simulink model "APA_AEB_Version_0_1"  (R2019a)
settings: Solver=FixedStepAuto  StartTime=0.0  StopTime=2  FixedStep=0.01  RelTol=1e-3
libraries: simulink x4, dspnetwork x1, autolibshared x1
(part 2 of 3)

== matlab function APA_AEB_Version_0_1/Ultarsonic Processment /Subsystem1/Subsystem1/MATLAB Function ==
  data: front_leftSide_uss_dist input single; front_leftFront_uss_dist input single; front_leftMiddle_uss_dist input single; front_rightMiddle_uss_dist input single; front_rightFront_uss_dist input single; front_rightSide_uss_dist input single; rear_leftSide_uss_dist input single; rear_leftRear_uss_dist input single; rear_leftMiddle_uss_dist input single; rear_rightMiddle_uss_dist input single; rear_rightRear_uss_dist input single; Useful_flag output single; Front_Object_dist_x output single; Front_Object_dist_y output single; Rear_Object_dist_x output single; Rear_Object_dist_y output single; rear_rightSide_uss_dist input single; USS_Position input single
function [ Useful_flag,Front_Object_dist_x,Front_Object_dist_y,Rear_Object_dist_x,Rear_Object_dist_y]  = Obj_Position_Identify(front_leftSide_uss_dist,...
                                        front_leftFront_uss_dist,...
                                        front_leftMiddle_uss_dist,...
                                        front_rightMiddle_uss_dist,...
                                        front_rightFront_uss_dist,...
                                        front_rightSide_uss_dist,...
                                        rear_leftSide_uss_dist,...
                                        rear_leftRear_uss_dist,...
                                        rear_leftMiddle_uss_dist,...
                                        rear_rightMiddle_uss_dist,...
                                        rear_rightRear_uss_dist,...
                                        rear_rightSide_uss_dist,...
                                        USS_Position)
                                    
        USS_dist  = [single(360.6744),single(640.6000),single(360.6231),single(398.5876),single(560.8000),single(398.5876)];
        %
        USS_ID  = [single(0),single(0),single(0),single(0),single(0),single(0),single(0),single(0),single(0),single(0),single(0),single(0)];
        %
        Front_leftSide_uss_position_x  = single(3237.1);
        %
        Front_leftSide_uss_position_y  = single(-913.1);
        %
        Front_leftFront_uss_position_x  = single(3528.8);
        %
        Front_leftFront_uss_position_y  = single(-650.5);
        %
        Front_leftMiddle_uss_position_x  = single(3673.9);
        %
        Front_leftMiddle_uss_position_y  = single(-320.3);
        %
        Front_rightMiddle_uss_position_x  = single(3673.9);
        %
        Front_rightMiddle_uss_position_y  = single(320.3);
        %
        Front_rightFront_uss_position_x  =  single(3528.7);
        %
        Front_rightFront_uss_position_y  =  single(650.4);
        %
        Front_rightSide_uss_position_x  =  single(3337.1);
        %
        Front_rightSide_uss_position_y  =  single(913.1);
        %
        Rear_leftSide_uss_position_x  =  single(-432.3);
        %
        Rear_leftSide_uss_position_y  =  single(-915.1);
        %
        Rear_leftRear_uss_position_x  =  single(-784.2);
        %
        Rear_leftRear_uss_position_y  =  single(-660.4);
        %
        Rear_leftMiddle_uss_position_x  =  single(-904.5);
        %
        Rear_leftMiddle_uss_position_y  =  single(-280.4);
        %
        Rear_rightMiddle_uss_position_x  =  single(-904.5);
        %
        Rear_rightMiddle_uss_position_y  =  single(280.4);
        %
        Rear_rightRear_uss_position_x  =  single(-784.2);
        %
        Rear_rightRear_uss_position_y  =  single(660.4);
        %
        Rear_rightSide_uss_position_x  =  single(-432.3);
        %
        Rear_rightSide_uss_position_y  =  single(915.1);
        %
        Front_Object_dist_x  = [single(0),single(0),single(0),single(0),single(0)];
        %
        Front_Object_dist_y  = [single(0),single(0),single(0),single(0),single(0)];
        %
        Rear_Object_dist_x  = [single(0),single(0),single(0),single(0),single(0)];
        %
        Rear_Object_dist_y  = [single(0),single(0),single(0),single(0),single(0)];
        %
        Left_Object_dist_x  = [single(0),single(0),single(0),single(0),single(0)];
        %
        Left_Object_dist_y  = [single(0),single(0),single(0),single(0),single(0)];
        %
        Right_Object_dist_x  = [single(0),single(0),single(0),single(0),single(0)];
        %
        Right_Object_dist_y  = [single(0),single(0),single(0),single(0),single(0)];
        %
        point_num  = single(5);
        %
        Front_leftSide_uss_FOV  = [single(0.9986),single(0.0523);single(0.0523),single(-0.9986)];
        %
        Front_leftSide_uss_FOV_theta_min  = single(3*single(3.141593/4));
        %
        Front_leftSide_uss_FOV_theta_max  = single(3.141593/4);
        %
        Front_leftFront_uss_FOV  = [single(0.6252),single(0.7804);single(0.7804),single(-0.6252)];
        %
        Front_leftFront_uss_FOV_theta_min  = single(3*single(3.141593/4));
        %
        Front_leftFront_uss_FOV_theta_max  = single(3.141593/4);
        %
        Front_leftMiddle_uss_FOV  = [single(0.3190),single(0.9478);single(0.9478),single(-0.3190)];
        %
        Front_leftMiddle_uss_FOV_theta_min  = single(3*single(3.141593/4));
        %
        Front_leftMiddle_uss_FOV_theta_max  = single(3.141593/4);
        %
        Front_rightMiddle_uss_FOV  = [single(-0.3190),single(0.9478);single(0.9478),single(0.3190)];
        %
        Front_rightMiddle_uss_FOV_theta_min  = single(3*single(3.141593/4));
        %
        Front_rightMiddle_uss_FOV_theta_max  = single(3.141593/4);
        %
        Front_rightFront_uss_FOV  = [single(-0.6252),single(0.7804);single(0.7804),single(0.6252)];
        %
        Front_rightFront_uss_FOV_theta_min  = single(3*single(3.141593/4));
        %
        Front_rightFront_uss_FOV_theta_max  = single(3.141593/4);
        %
        Front_rightSide_uss_FOV  = [single(-0.9986),single(0.0523);single(0.0523),single(0.9986)];
        %
        Front_rightSide_uss_FOV_theta_min  = single(3*single(3.141593/4));
        %
        Front_rightSide_uss_FOV_theta_max  = single(3.141593/4);
        %
        Rear_leftSide_uss_FOV  = [single(0.9986),single(-0.0523);single(-0.0523),single(-0.9986)];
        %
        Rear_leftSide_uss_FOV_theta_min  = single(3*single(3.141593/4));
        %
        Rear_leftSide_uss_FOV_theta_max  = single(3.141593/4);
        %
        Rear_leftRear_uss_FOV  = [single(0.4602),single(-0.8878);single(-0.8878),single(-0.4602)];
        %
        Rear_leftRear_uss_FOV_theta_min  = single(3*single(3.141593/4));
        %
        Rear_leftRear_uss_FOV_theta_max  = single(3.141593/4);
        %
        Rear_leftMiddle_uss_FOV  = [single(0.1097),single(-0.9940);single(-0.9940),single(-0.1097)];
        %
        Rear_leftMiddle_uss_FOV_theta_min  = single(3*single(3.141593/4));
        %
        Rear_leftMiddle_uss_FOV_theta_max  = single(3.141593/4);
        %
        Rear_rightMiddle_uss_FOV  = [single(-0.1097),single(-0.9940);single(-0.9940),single(0.1097)];
        %
        Rear_rightMiddle_uss_FOV_theta_min  = single(3*single(3.141593/4));
        %
        Rear_rightMiddle_uss_FOV_theta_max  = single(3.141593/4);
        %
        Rear_rightRear_uss_FOV  = [single(-0.4602),single(-0.8878);single(-0.8878),single(0.4602)];
        %
        Rear_rightRear_uss_FOV_theta_min  = single(3*single(3.141593/4));
        %
        Rear_rightRear_uss_FOV_theta_max  = single(3.141593/4);
        %
        Rear_rightSide_uss_FOV  = [single(-0.9986),single(-0.0523);single(-0.0523),single(0.9986)];
        %
        Rear_rightSide_uss_FOV_theta_min  = single(3*single(3.141593/4));
        %
        Rear_rightSide_uss_FOV_theta_max  = single(3.141593/4);
        %
        USS_Location_Left  = single(0);
        %
        USS_Location_Right  = single(0);
        %
        USS_Location  = single(0);
        %
        front_dist  = [single(0),single(0),single(0),single(0)];
        %
        Rear_dist  = [single(0),single(0),single(0),single(0)];
        %
        alpha  = single(0);
        %
        front_min  = single(0);
        %
        front_flag  = single(0);
        %
        Rear_min  = single(0);
        %
        rear_flag  = single(0);
        %
        Front_Position_flag  = single(0);
        %
        Rear_Position_flag  = single(0);
        %
        gap = single(3.141593/8);
        %
        theta = single(3.141593.*[3/4, 5/8, 1/2, 3/8, 1/4]) ;
        %
        theta_far = single(3.141593.*[5/8, 9/16, 1/2, 7/16, 3/8]);
        %
        theta_side = single(3.141593.*[42/72, 39/72, 36/72, 33/72, 30/72]);
        %
        Useful_flag = single(0);
        %
        if front_leftSide_uss_dist == single(0) && rear_leftSide_uss_dist == single(0)
            Left_Object_dist_x = single([0,0,0,0,0]);
            Left_Object_dist_y = single([0,0,0,0,0]);
        elseif front_leftSide_uss_dist > single(0) && rear_leftSide_uss_dist == single(0)
            USS_ID(1)=single(1);
        elseif front_leftSide_uss_dist == single(0) && rear_leftSide_uss_dist > single(0)
            USS_ID(7)=single(1);
        elseif front_leftSide_uss_dist > single(0) && rear_leftSide_uss_dist > single(0)
               if front_leftSide_uss_dist < rear_leftSide_uss_dist || front_leftSide_uss_dist == rear_leftSide_uss_dist
                    USS_ID(1) = single(1);
               else
                    USS_ID(7) = single(1);
               end
        end

        if  front_rightSide_uss_dist == single(0) && rear_rightSide_uss_dist == single(0)
            Right_Object_dist_x = single([0,0,0,0,0]);
            Right_Object_dist_y = single([0,0,0,0,0]);
        elseif front_rightSide_uss_dist > single(0) && rear_rightSide_uss_dist == single(0)
            USS_ID(6)=single(1);
        elseif front_rightSide_uss_dist == single(0) && rear_rightSide_uss_dist > single(0)
            USS_ID(12)=single(1);
        elseif front_rightSide_uss_dist > single(0) && rear_rightSide_uss_dist > single(0)
            if front_rightSide_uss_dist < rear_rightSide_uss_dist || front_rightSide_uss_dist == rear_rightSide_uss_dist
                    USS_ID(6) = single(1);
            else
                    USS_ID(12) = single(1);
            end
        end
        if front_leftFront_uss_dist == single(0) && front_leftMiddle_uss_dist == single(0) && front_rightMiddle_uss_dist == single(0) && front_rightFront_uss_dist == single(0)
            Front_Position_flag = single(0);
        else
            front_dist=single([front_leftFront_uss_dist,front_leftMiddle_uss_dist,front_rightMiddle_uss_dist,front_rightFront_uss_dist]);
           if front_dist(1)>single(0)&&front_dist(2)==single(0)&&front_dist(3)==single(0)&&front_dist(4)==single(0)
               front_min = front_dist(1);
           elseif front_dist(1)==single(0)&&front_dist(2)>single(0)&&front_dist(3)==single(0)&&front_dist(4)==single(0)
               front_min = front_dist(2);
           elseif front_dist(1)==single(0)&&front_dist(2)==single(0)&&front_dist(3)>single(0)&&front_dist(4)==single(0)
               front_min = front_dist(3);
           elseif front_dist(1)==single(0)&&front_dist(2)==single(0)&&front_dist(3)==single(0)&&front_dist(4)>single(0)
               front_min = front_dist(4);
           elseif front_dist(1)>single(0)&&front_dist(2)>single(0)&&front_dist(3)==single(0)&&front_dist(4)==single(0)
               front_min = min( single([front_dist(1), front_dist(2)]));
           elseif front_dist(1)>single(0)&&front_dist(2)==single(0)&&front_dist(3)>single(0)&&front_dist(4)==single(0)
               front_min = min( single([front_dist(1), front_dist(3)]));
           elseif front_dist(1)==single(0)&&front_dist(2)>single(0)&&front_dist(3)>single(0)&&front_dist(4)==single(0)
               front_min = min( single([front_dist(2), front_dist(3)]));
           elseif front_dist(1)==single(0)&&front_dist(2)>single(0)&&front_dist(3)==single(0)&&front_dist(4)>single(0)
               front_min = min( single([front_dist(2), front_dist(4)]));
           elseif front_dist(1)==single(0)&&front_dist(2)==single(0)&&front_dist(3)>single(0)&&front_dist(4)>single(0)
               front_min = min( single([front_dist(3), front_dist(4)]));
           elseif front_dist(1)>single(0)&&front_dist(2)==single(0)&&front_dist(3)==single(0)&&front_dist(4)>single(0)
               front_min = min( single([front_dist(1), front_dist(4)]));
           elseif front_dist(1)>single(0)&&front_dist(2)>single(0)&&front_dist(3)>single(0)&&front_dist(4)==single(0)
               front_min = min( single([front_dist(1), front_dist(2),front_dist(3)]));
           elseif front_dist(1)>single(0)&&front_dist(2)>single(0)&&front_dist(3)==single(0)&&front_dist(4)>single(0)
               front_min = min(single([ front_dist(1), front_dist(2),front_dist(4)]));
           elseif front_dist(1)>single(0)&&front_dist(2)==single(0)&&front_dist(3)>single(0)&&front_dist(4)>single(0)
               front_min = min(single([ front_dist(1), front_dist(3),front_dist(4)]));
           elseif front_dist(1)==single(0)&&front_dist(2)>single(0)&&front_dist(3)>single(0)&&front_dist(4)>single(0)
               front_min = min( single([front_dist(2), front_dist(3),front_dist(4)]));
           elseif front_dist(1)>single(0)&&front_dist(2)>single(0)&&front_dist(3)>single(0)&&front_dist(4)>single(0)
               front_min = min( single([front_dist(1), front_dist(2),front_dist(3),front_dist(4)]));        
           end
                if front_min == front_dist(1)
                    if front_dist(2)> single(0) && front_dist(3) == single(0) && front_dist(1)+front_dist(2)> USS_dist(1)                     
                        Front_Position_flag = single(1);
                    else 
                         Front_Position_flag = single(0);
                         USS_ID(2)=single(1);
                    end
                elseif front_min == front_dist(2)
                    if front_dist(1)> single(0) && front_dist(3) == single(0)&& front_dist(1)+front_dist(2)> USS_dist(1)
                        Front_Position_flag = single(1);
                    elseif front_dist(1)== single(0) && front_dist(3) > single(0) && front_dist(4) == single(0)&& front_dist(3)+front_dist(2)> USS_dist(2)
                        Front_Position_flag = single(2);
                    else
                        Front_Position_flag = single(0);
                        USS_ID(3)=single(1);
                    end
                elseif front_min == front_dist(3)
                    if front_dist(2)> single(0) && front_dist(4) == single(0) && front_dist(1) == single(0)&& front_dist(3)+front_dist(2)> USS_dist(2)
                        Front_Position_flag = single(2);
                    elseif front_dist(2)== single(0) && front_dist(4) > single(0)&&front_dist(3)+front_dist(4)> USS_dist(3)
                        Front_Position_flag = single(3);
                    else
                        Front_Position_flag = single(0);
                        USS_ID(4)=single(1);
                    end
                elseif front_min == front_dist(4)
                    if front_dist(3)> single(0) && front_dist(2) == single(0)&&front_dist(3)+front_dist(4)> USS_dist(3)                         
                        Front_Position_flag = single(3);
                    else
                         Front_Position_flag = single(0);
                         USS_ID(5)=single(1);
                    end
                end
        end

        if rear_leftRear_uss_dist == single(0) && rear_leftMiddle_uss_dist == single(0) && rear_rightMiddle_uss_dist == single(0) && rear_rightRear_uss_dist == single(0)
            Rear_Position_flag  = single(single(0));
        else
            Rear_dist=single([rear_leftRear_uss_dist,rear_leftMiddle_uss_dist,rear_rightMiddle_uss_dist,rear_rightRear_uss_dist]);
           if Rear_dist(1)>single(0)&&Rear_dist(2)==single(0)&&Rear_dist(3)==single(0)&&Rear_dist(4)==single(0)
               Rear_min = Rear_dist(1);
           elseif Rear_dist(1)==single(0)&&Rear_dist(2)>single(0)&&Rear_dist(3)==single(0)&&Rear_dist(4)==single(0)
               Rear_min = Rear_dist(2);
           elseif Rear_dist(1)==single(0)&&Rear_dist(2)==single(0)&&Rear_dist(3)>single(0)&&Rear_dist(4)==single(0)
               Rear_min = Rear_dist(3);
           elseif Rear_dist(1)==single(0)&&Rear_dist(2)==single(0)&&Rear_dist(3)==single(0)&&Rear_dist(4)>single(0)
               Rear_min = Rear_dist(4);
           elseif Rear_dist(1)>single(0)&&Rear_dist(2)>single(0)&&Rear_dist(3)==single(0)&&Rear_dist(4)==single(0)
               Rear_min = min( single([Rear_dist(1), Rear_dist(2)]));
           elseif Rear_dist(1)>single(0)&&Rear_dist(2)==single(0)&&Rear_dist(3)>single(0)&&Rear_dist(4)==single(0)
               Rear_min = min( single([Rear_dist(1), Rear_dist(3)]));
           elseif Rear_dist(1)==single(0)&&Rear_dist(2)>single(0)&&Rear_dist(3)>single(0)&&Rear_dist(4)==single(0)
               Rear_min = min( single([Rear_dist(2), Rear_dist(3)]));
           elseif Rear_dist(1)==single(0)&&Rear_dist(2)>single(0)&&Rear_dist(3)==single(0)&&Rear_dist(4)>single(0)
               Rear_min = min( single([Rear_dist(2), Rear_dist(4)]));
           elseif Rear_dist(1)==single(0)&&Rear_dist(2)==single(0)&&Rear_dist(3)>single(0)&&Rear_dist(4)>single(0)
               Rear_min = min( single([Rear_dist(3), Rear_dist(4)]));
           elseif Rear_dist(1)>single(0)&&Rear_dist(2)==single(0)&&Rear_dist(3)==single(0)&&Rear_dist(4)>single(0)
               Rear_min = min( single([Rear_dist(1), Rear_dist(4)]));
           elseif Rear_dist(1)>single(0)&&Rear_dist(2)>single(0)&&Rear_dist(3)>single(0)&&Rear_dist(4)==single(0)
               Rear_min = min( single([Rear_dist(1), Rear_dist(2),Rear_dist(3)]));
           elseif Rear_dist(1)>single(0)&&Rear_dist(2)>single(0)&&Rear_dist(3)==single(0)&&Rear_dist(4)>single(0)
               Rear_min = min(single([ Rear_dist(1), Rear_dist(2),Rear_dist(4)]));
           elseif Rear_dist(1)>single(0)&&Rear_dist(2)==single(0)&&Rear_dist(3)>single(0)&&Rear_dist(4)>single(0)
               Rear_min = min(single([ Rear_dist(1), Rear_dist(3),Rear_dist(4)]));
           elseif Rear_dist(1)==single(0)&&Rear_dist(2)>single(0)&&Rear_dist(3)>single(0)&&Rear_dist(4)>single(0)
               Rear_min = min( single([Rear_dist(2), Rear_dist(3),Rear_dist(4)]));
           elseif Rear_dist(1)>single(0)&&Rear_dist(2)>single(0)&&Rear_dist(3)>single(0)&&Rear_dist(4)>single(0)
               Rear_min = min( single([Rear_dist(1), Rear_dist(2),Rear_dist(3),Rear_dist(4)]));        
           end
            if Rear_min == Rear_dist(1)
                    if Rear_dist(2)> single(0) && Rear_dist(3) == single(0)&&Rear_dist(1)+Rear_dist(2)> USS_dist(4)                           
                        Rear_Position_flag = single(1);
                    else
                         Rear_Position_flag = single(0);
                         USS_ID(8) = single(1);
                    end
            elseif Rear_min == Rear_dist(2)
                    if Rear_dist(1)> single(0) && Rear_dist(3) == single(0)&&Rear_dist(1)+Rear_dist(2)> USS_dist(4)
                        Rear_Position_flag = single(1);
                    elseif Rear_dist(1)== single(0) && Rear_dist(3) > single(0) && Rear_dist(4) == single(0)&&Rear_dist(3)+Rear_dist(2)> USS_dist(5)
                        Rear_Position_flag = single(2);
                    else
                        Rear_Position_flag =single(0);
                        USS_ID(9) = single(1);
                    end
            elseif Rear_min == Rear_dist(3)
                    if Rear_dist(2)> single(0) && Rear_dist(4) == single(0) && Rear_dist(1) == single(0)&&Rear_dist(3)+Rear_dist(2)> USS_dist(5)
                        Rear_Position_flag = single(2);
                    elseif Rear_dist(2)== single(0) && Rear_dist(4) > single(0)&&Rear_dist(3)+Rear_dist(4)> USS_dist(6)
                        Rear_Position_flag = single(3);
                    else
                        Rear_Position_flag = single(0);
                        USS_ID(10)=single(1);
                    end
             elseif Rear_min == Rear_dist(4)
                    if Rear_dist(3)> single(0) && Rear_dist(2) == single(0)&&Rear_dist(3)+Rear_dist(4)> USS_dist(6)                           
                        Rear_Position_flag = single(3);
                    else
                         Rear_Position_flag = single(0);
                         USS_ID(11)=single(1);
                    end
            end       
        end
        
        if Front_Position_flag == single(0) || Rear_Position_flag == single(0)
            for num = single(1:12)
            if USS_ID(num)==single(1)
                switch num
                    case single(1)
                        USS_Location = front_leftSide_uss_dist;
                        orix = USS_Location * single(cos(theta_side));
                        oriy = sqrt(USS_Location^2-orix.^2);
                        Left_Object_dist_x = orix.* Front_leftSide_uss_FOV(1,1) + oriy.*Front_leftSide_uss_FOV(2,1) + Front_leftSide_uss_position_x;
                        Left_Object_dist_y = orix.* Front_leftSide_uss_FOV(1,2) + oriy.*Front_leftSide_uss_FOV(2,2) + Front_leftSide_uss_position_y;
                    case single(2)
                        USS_Location=front_leftFront_uss_dist;
                        if USS_Location <= 600
                            orix = USS_Location * cos(theta);
                        else
                            orix = USS_Location * cos(theta_far);
                        end
                        oriy = sqrt(USS_Location^2-orix.^2);
                        Front_Object_dist_x = orix.* Front_leftFront_uss_FOV(1,1) + oriy.*Front_leftFront_uss_FOV(2,1) + Front_leftFront_uss_position_x;
                        Front_Object_dist_y = orix.* Front_leftFront_uss_FOV(1,2) + oriy.*Front_leftFront_uss_FOV(2,2) + Front_leftFront_uss_position_y;
                    case single(3)
                        USS_Location=front_leftMiddle_uss_dist;
                        if USS_Location <= 600
                            orix = USS_Location * cos(theta);
                        else
                            orix = USS_Location * cos(theta_far);
                        end
                        oriy = sqrt(USS_Location^2-orix.^2);
                        Front_Object_dist_x = orix.* Front_leftMiddle_uss_FOV(1,1) + oriy.*Front_leftMiddle_uss_FOV(2,1) + Front_leftMiddle_uss_position_x;
                        Front_Object_dist_y = orix.* Front_leftMiddle_uss_FOV(1,2) + oriy.*Front_leftMiddle_uss_FOV(2,2) + Front_leftMiddle_uss_position_y;
                    case single(4)
                        USS_Location=front_rightMiddle_uss_dist;
                        if USS_Location <= 600
                            orix = USS_Location * cos(theta);
                        else
                            orix = USS_Location * cos(theta_far);
                        end
                        oriy = sqrt(USS_Location^2-orix.^2);
                        Front_Object_dist_x = orix.* Front_rightMiddle_uss_FOV(1,1) + oriy.*Front_rightMiddle_uss_FOV(2,1) + Front_rightMiddle_uss_position_x;
                        Front_Object_dist_y = orix.* Front_rightMiddle_uss_FOV(1,2) + oriy.*Front_rightMiddle_uss_FOV(2,2) + Front_rightMiddle_uss_position_y;
                    case single(5)
                        USS_Location=front_rightFront_uss_dist;
                        if USS_Location <= 600
                            orix = USS_Location * cos(theta);
                        else
                            orix = USS_Location * cos(theta_far);
                        end
                        oriy = sqrt(USS_Location^2-orix.^2);
                        Front_Object_dist_x = orix.* Front_rightFront_uss_FOV(1,1) + oriy.*Front_rightFront_uss_FOV(2,1) + Front_rightFront_uss_position_x;
                        Front_Object_dist_y = orix.* Front_rightFront_uss_FOV(1,2) + oriy.*Front_rightFront_uss_FOV(2,2) + Front_rightFront_uss_position_y;
                    case single(6)
                        USS_Location=front_rightSide_uss_dist;
                        orix = USS_Location * cos(theta_side);
                        oriy = sqrt(USS_Location^2-orix.^2);
                        Right_Object_dist_x = orix.* Front_rightSide_uss_FOV(1,1) + oriy.*Front_rightSide_uss_FOV(2,1) + Front_rightSide_uss_position_x;
                        Right_Object_dist_y = orix.* Front_rightSide_uss_FOV(1,2) + oriy.*Front_rightSide_uss_FOV(2,2) + Front_rightSide_uss_position_y;
                    case single(7)
                        USS_Location=rear_leftSide_uss_dist;
                        orix = USS_Location * cos(theta_side);
                        oriy = sqrt(USS_Location^2-orix.^2);
                        Left_Object_dist_x = orix.* Rear_leftSide_uss_FOV(1,1) + oriy.*Rear_leftSide_uss_FOV(2,1) + Rear_leftSide_uss_position_x;
                        Left_Object_dist_y = orix.* Rear_leftSide_uss_FOV(1,2) + oriy.*Rear_leftSide_uss_FOV(2,2) + Rear_leftSide_uss_position_y;
                    case single(8)
                        USS_Location=rear_leftRear_uss_dist;
                        if USS_Location <= 600
                            orix = USS_Location * cos(theta);
                        else
                            orix = USS_Location * cos(theta_far);
                        end
                        oriy = sqrt(USS_Location^2-orix.^2);
                        Rear_Object_dist_x = orix.* Rear_leftRear_uss_FOV(1,1) + oriy.*Rear_leftRear_uss_FOV(2,1) + Rear_leftRear_uss_position_x;
                        Rear_Object_dist_y = orix.* Rear_leftRear_uss_FOV(1,2) + oriy.*Rear_leftRear_uss_FOV(2,2) + Rear_leftRear_uss_position_y;
                    case single(9)
                        USS_Location=rear_leftMiddle_uss_dist;
                        if USS_Location <= 600
                            orix = USS_Location * cos(theta);
                        else
                            orix = USS_Location * cos(theta_far);
                        end
                        oriy = sqrt(USS_Location^2-orix.^2);
                        Rear_Object_dist_x = orix.* Rear_leftMiddle_uss_FOV(1,1) + oriy.*Rear_leftMiddle_uss_FOV(2,1) + Rear_leftMiddle_uss_position_x;
                        Rear_Object_dist_y = orix.* Rear_leftMiddle_uss_FOV(1,2) + oriy.*Rear_leftMiddle_uss_FOV(2,2) + Rear_leftMiddle_uss_position_y;
                    case single(10)
                        USS_Location=rear_rightMiddle_uss_dist;
                        if USS_Location <= 600
                            orix = USS_Location * cos(theta);
                        else
                            orix = USS_Location * cos(theta_far);
                        end
                        oriy = sqrt(USS_Location^2-orix.^2);
                        Rear_Object_dist_x = orix.* Rear_rightMiddle_uss_FOV(1,1) + oriy.*Rear_rightMiddle_uss_FOV(2,1) + Rear_rightMiddle_uss_position_x;
                        Rear_Object_dist_y = orix.* Rear_rightMiddle_uss_FOV(1,2) + oriy.*Rear_rightMiddle_uss_FOV(2,2) + Rear_rightMiddle_uss_position_y;
                    case single(11)
                        USS_Location=rear_rightRear_uss_dist;
                        if USS_Location <= 600
                            orix = USS_Location * cos(theta);
                        else
                            orix = USS_Location * cos(theta_far);
                        end
                        oriy = sqrt(USS_Location^2-orix.^2);
                        Rear_Object_dist_x = orix.* Rear_rightRear_uss_FOV(1,1) + oriy.*Rear_rightRear_uss_FOV(2,1) + Rear_rightRear_uss_position_x;
                        Rear_Object_dist_y = orix.* Rear_rightRear_uss_FOV(1,2) + oriy.*Rear_rightRear_uss_FOV(2,2) + Rear_rightRear_uss_position_y;
                    case single(12)
                        USS_Location=rear_rightSide_uss_dist;
                        orix = USS_Location * cos(theta_side);
                        oriy = sqrt(USS_Location^2-orix.^2);
                        Right_Object_dist_x = orix.* Rear_rightSide_uss_FOV(1,1) + oriy.*Rear_rightSide_uss_FOV(2,1) + Rear_rightSide_uss_position_x;
                        Right_Object_dist_y = orix.* Rear_rightSide_uss_FOV(1,2) + oriy.*Rear_rightSide_uss_FOV(2,2) + Rear_rightSide_uss_position_y;
                end
            end
            end
        end
        if Front_Position_flag == single(1)
            %
            USS_Location_Left = front_leftFront_uss_dist;
            %
            USS_Location_Right = front_leftMiddle_uss_dist;
            %
            alpha = single(acos((USS_dist(1)^2+USS_Location_Left^2-USS_Location_Right^2)/(2 * USS_dist(1) * USS_Location_Left)));
            %
            x = single(sin(alpha)*USS_Location_Left);
            %
            y = single(cos(alpha)*USS_Location_Left); 
            %
            a = (Front_leftMiddle_uss_position_x - Front_leftFront_uss_position_x)/USS_dist(1);
            %
            b= abs(Front_leftMiddle_uss_position_y - Front_leftFront_uss_position_y)/USS_dist(1);
            %
            Front_Object_dist_x(1) = x * b + y * a + Front_leftFront_uss_position_x;
            %
            Front_Object_dist_y(1) = - x * a + y * b + Front_leftFront_uss_position_y;
            %
            Useful_flag = single(1);
            %
        elseif Front_Position_flag == 2
            %
            USS_Location_Left = front_leftMiddle_uss_dist;
            %
            USS_Location_Right = front_rightMiddle_uss_dist;
            %
            alpha = acos((USS_dist(2)^2+USS_Location_Left^2-USS_Location_Right^2)/(2 * USS_dist(2) * USS_Location_Left));
            %
            x = sin(alpha)*USS_Location_Left;
            %
            y = cos(alpha)*USS_Location_Left;
            %
            a = (Front_rightMiddle_uss_position_x - Front_leftMiddle_uss_position_x)/USS_dist(2);
            %
            b = abs(Front_rightMiddle_uss_position_y - Front_leftMiddle_uss_position_y)/USS_dist(2);
            %
            Front_Object_dist_x(1) = x * b + y * a + Front_leftMiddle_uss_position_x;
            %
            Front_Object_dist_y(1) = - x * a + y * b + Front_leftMiddle_uss_position_y;
            %
            Useful_flag = single(1);
            %
        elseif Front_Position_flag == 3
            %
            USS_Location_Left = front_rightMiddle_uss_dist;
            %
            USS_Location_Right = front_rightFront_uss_dist;
            %
            alpha = acos((USS_dist(3)^2+USS_Location_Left^2-USS_Location_Right^2)/(2 * USS_dist(3) * USS_Location_Left));
            %
            Front_Object_dist_x(1) = sin(alpha)*USS_Location_Left+Front_rightMiddle_uss_position_x;
            %
            Front_Object_dist_y(1) = cos(alpha)*USS_Location_Left+Front_rightMiddle_uss_position_y;
            %
            x = sin(alpha)*USS_Location_Left;
            %
            y = cos(alpha)*USS_Location_Left;
            %
            a = (Front_rightFront_uss_position_x - Front_rightMiddle_uss_position_x)/USS_dist(3);
            %
            b = abs(Front_rightFront_uss_position_y - Front_rightMiddle_uss_position_y)/USS_dist(3);
            %
            Front_Object_dist_x(1) = x * b + y * a + Front_rightMiddle_uss_position_x;
            %
            Front_Object_dist_y(1) = - x * a + y * b + Front_rightMiddle_uss_position_y;
            %
            Useful_flag = single(1);
            %
        end
            if Rear_Position_flag == 1
                %
                USS_Location_Left = rear_leftMiddle_uss_dist;
                %
                USS_Location_Right = rear_leftRear_uss_dist;
                %
                alpha = acos((USS_dist(4)^2+USS_Location_Left^2-USS_Location_Right^2)/(2 * USS_dist(4) * USS_Location_Left));
                %
                x = sin(alpha)*USS_Location_Left;
                %
                y = cos(alpha)*USS_Location_Left; 
                %
                a = -(Rear_leftRear_uss_position_x - Rear_leftMiddle_uss_position_x)/USS_dist(4);
                %
                b= abs(Rear_leftRear_uss_position_y - Rear_leftMiddle_uss_position_y)/USS_dist(4);
                %
                Rear_Object_dist_x(1) = - ( x * b + y * a ) + Rear_leftMiddle_uss_position_x;
                %
                Rear_Object_dist_y(1) = - ( - x * a + y * b ) + Rear_leftMiddle_uss_position_y;
                %
                Useful_flag = single(1);
                %
            elseif Rear_Position_flag == 2
                %
                USS_Location_Left = rear_rightMiddle_uss_dist;
                %
                USS_Location_Right = rear_leftMiddle_uss_dist;
                %
                alpha = acos((USS_dist(5)^2+USS_Location_Left^2-USS_Location_Right^2)/(2 * USS_dist(5) * USS_Location_Left));
                %
                x = sin(alpha)*USS_Location_Left;
                %
                y = cos(alpha)*USS_Location_Left; 
                %
                a = -(Rear_leftMiddle_uss_position_x - Rear_rightMiddle_uss_position_x)/USS_dist(5);
                %
                b= abs(Rear_leftMiddle_uss_position_y - Rear_rightMiddle_uss_position_y)/USS_dist(5);
                %
                Rear_Object_dist_x(1) = - ( x * b + y * a ) + Rear_rightMiddle_uss_position_x;
                %
                Rear_Object_dist_y(1) = - ( x * a + y * b ) + Rear_rightMiddle_uss_position_y;
                %
                Useful_flag = single(1);
                %
            elseif Rear_Position_flag == 3
                %
                USS_Location_Left = rear_rightRear_uss_dist;
                %
                USS_Location_Right = rear_rightMiddle_uss_dist;
                %
                alpha = acos((USS_dist(6)^2+USS_Location_Left^2-USS_Location_Right^2)/(2 * USS_dist(6) * USS_Location_Left));
                %
                x = sin(alpha) * USS_Location_Left;
                %
                y = cos(alpha )* USS_Location_Left; 
                %
                a = -(Rear_rightMiddle_uss_position_x - Rear_rightRear_uss_position_x)/USS_dist(6);
                %
                b= abs(Rear_rightMiddle_uss_position_y - Rear_rightRear_uss_position_y)/USS_dist(6);
                %
                Rear_Object_dist_x(1) = - ( x * b + y * a ) + Rear_rightRear_uss_position_x;
                %
                Rear_Object_dist_y(1) = - ( - x * a + y * b ) + Rear_rightRear_uss_position_y;
                %
                Useful_flag = single(1);
            end

== matlab function APA_AEB_Version_0_1/Ultarsonic Processment /Subsystem1/Subsystem1/Obj_Position_Identify ==
  settings: updateMethod=DISCRETE
  data: Sensor_Detection input single; Aera_Case_flag output single; Err_USS input single
function Aera_Case_flag  = Obj_Position_Identify(Sensor_Detection,Err_USS)

persistent Obj_Pos_flag

if isempty(Obj_Pos_flag)
    Obj_Pos_flag = 0;
end

if sum(Sensor_Detection)<Err_USS
    Obj_Pos_flag = 0;
elseif abs(Sensor_Detection(1) - sum(Sensor_Detection)) < Err_USS
    Obj_Pos_flag = 1;
elseif abs(Sensor_Detection(2) - sum(Sensor_Detection)) < Err_USS
    Obj_Pos_flag = 2;
elseif abs(Sensor_Detection(3) - sum(Sensor_Detection)) < Err_USS
    Obj_Pos_flag = 3;
elseif abs(Sensor_Detection(4) - sum(Sensor_Detection)) < Err_USS
    Obj_Pos_flag = 4;
elseif abs(Sensor_Detection(5) - sum(Sensor_Detection)) < Err_USS
    Obj_Pos_flag = 5;
elseif abs(Sensor_Detection(6) - sum(Sensor_Detection)) < Err_USS
    Obj_Pos_flag = 6;   
elseif abs(Sensor_Detection(7) - sum(Sensor_Detection)) < Err_USS
    Obj_Pos_flag = 7;   
elseif abs(Sensor_Detection(8) - sum(Sensor_Detection)) < Err_USS
    Obj_Pos_flag = 8;     
elseif abs(Sensor_Detection(9) - sum(Sensor_Detection)) < Err_USS
    Obj_Pos_flag = 9;  
elseif abs(Sensor_Detection(10) - sum(Sensor_Detection)) < Err_USS
    Obj_Pos_flag = 10;
elseif abs(Sensor_Detection(11) - sum(Sensor_Detection)) < Err_USS
    Obj_Pos_flag = 11; 
elseif abs(Sensor_Detection(12) - sum(Sensor_Detection)) < Err_USS
    Obj_Pos_flag = 12; 
elseif abs(Sensor_Detection(1) + Sensor_Detection(2) - sum(Sensor_Detection)) < Err_USS
    Obj_Pos_flag = 13;
elseif abs(Sensor_Detection(2) + Sensor_Detection(3) - sum(Sensor_Detection)) < Err_USS
    Obj_Pos_flag = 14;
elseif abs(Sensor_Detection(3) + Sensor_Detection(4) - sum(Sensor_Detection)) < Err_USS
    Obj_Pos_flag = 15;
elseif abs(Sensor_Detection(4) + Sensor_Detection(5) - sum(Sensor_Detection)) < Err_USS
    Obj_Pos_flag = 16;
elseif abs(Sensor_Detection(5) + Sensor_Detection(6) - sum(Sensor_Detection)) < Err_USS
    Obj_Pos_flag = 17; 
elseif abs(Sensor_Detection(6) + Sensor_Detection(7) - sum(Sensor_Detection)) < Err_USS
    Obj_Pos_flag = 18;
elseif abs(Sensor_Detection(7) + Sensor_Detection(8) - sum(Sensor_Detection)) < Err_USS
    Obj_Pos_flag = 19;
elseif abs(Sensor_Detection(8) + Sensor_Detection(9) - sum(Sensor_Detection)) < Err_USS
    Obj_Pos_flag = 20;
elseif abs(Sensor_Detection(9) + Sensor_Detection(10) - sum(Sensor_Detection)) < Err_USS
    Obj_Pos_flag = 21;
elseif abs(Sensor_Detection(10) + Sensor_Detection(11) - sum(Sensor_Detection)) < Err_USS
    Obj_Pos_flag = 22;
elseif abs(Sensor_Detection(11) + Sensor_Detection(12) - sum(Sensor_Detection)) < Err_USS
    Obj_Pos_flag = 23;
elseif abs(Sensor_Detection(12) + Sensor_Detection(1) - sum(Sensor_Detection)) < Err_USS
    Obj_Pos_flag = 24;
else
    Obj_Pos_flag = 25;
end
    
Aera_Case_flag = single(Obj_Pos_flag);

== matlab function APA_AEB_Version_0_1/Ultarsonic Processment /Subsystem1/Subsystem1/Find_Obj_USS_ID ==
  data: Detection_ID output single size=[12 12]; Sensor_Detection input single; Blind_Err input single; Detect_Sum output single
function [Detection_ID, Detect_Sum]  = Find_Obj_USS_ID(Sensor_Detection,Blind_Err)
% Detection_ID = zeros(1,12);
% coder.varsize('Detection_ID');
Detection_ID = find(Sensor_Detection>Blind_Err);

Detect_Sum = length(Detection_ID);

== matlab function APA_AEB_Version_0_1/Ultarsonic Processment /Subsystem1/Subsystem1/Detection Processment/Switch Case Action Subsystem/MATLAB Function ==
  data: Sensor_Detection input; Longitudial_Dist output; Lateral_Dist output
function [Longitudial_Dist,Lateral_Dist] = fcn(Sensor_Detection)
    %
    Longitudial_Dist = single(zeros(5,12));
    %
    Lateral_Dist = single(zeros(5,12));
    %
    Front_leftSide_uss_position_x  = single(3237.1);
    %
    Front_leftSide_uss_position_y  = single(-913.1);
    %
    Front_leftFront_uss_position_x  = single(3528.8);
    %
    Front_leftFront_uss_position_y  = single(-650.5);
    %
    Front_leftMiddle_uss_position_x  = single(3673.9);
    %
    Front_leftMiddle_uss_position_y  = single(-320.3);
    %
    Front_rightMiddle_uss_position_x  = single(3673.9);
    %
    Front_rightMiddle_uss_position_y  = single(320.3);
    %
    Front_rightFront_uss_position_x  =  single(3528.7);
    %
    Front_rightFront_uss_position_y  =  single(650.4);
    %
    Front_rightSide_uss_position_x  =  single(3337.1);
    %
    Front_rightSide_uss_position_y  =  single(913.1);
    %
    Rear_leftSide_uss_position_x  =  single(-432.3);
    %
    Rear_leftSide_uss_position_y  =  single(-915.1);
    %
    Rear_leftRear_uss_position_x  =  single(-784.2);
    %
    Rear_leftRear_uss_position_y  =  single(-660.4);
    %
    Rear_leftMiddle_uss_position_x  =  single(-904.5);
    %
    Rear_leftMiddle_uss_position_y  =  single(-280.4);
    %
    Rear_rightMiddle_uss_position_x  =  single(-904.5);
    %
    Rear_rightMiddle_uss_position_y  =  single(280.4);
    %
    Rear_rightRear_uss_position_x  =  single(-784.2);
    %
    Rear_rightRear_uss_position_y  =  single(660.4);
    %
    Rear_rightSide_uss_position_x  =  single(-432.3);
    %
    Rear_rightSide_uss_position_y  =  single(915.1);
    %
    Front_leftSide_uss_FOV  = [single(0.9986),single(0.0523);single(0.0523),single(-0.9986)];
    %
    Front_leftFront_uss_FOV  = [single(0.6252),single(0.7804);single(0.7804),single(-0.6252)];
    %
    Front_leftMiddle_uss_FOV  = [single(0.3190),single(0.9478);single(0.9478),single(-0.3190)];
    %
    Front_rightMiddle_uss_FOV  = [single(-0.3190),single(0.9478);single(0.9478),single(0.3190)];
    %
    Front_rightFront_uss_FOV  = [single(-0.6252),single(0.7804);single(0.7804),single(0.6252)];
    %
    Front_rightSide_uss_FOV  = [single(-0.9986),single(0.0523);single(0.0523),single(0.9986)];
    %
    Rear_leftSide_uss_FOV  = [single(0.9986),single(-0.0523);single(-0.0523),single(-0.9986)];
    %
    Rear_leftRear_uss_FOV  = [single(0.4602),single(-0.8878);single(-0.8878),single(-0.4602)];
    %
    Rear_leftMiddle_uss_FOV  = [single(0.1097),single(-0.9940);single(-0.9940),single(-0.1097)];
    %
    Rear_rightMiddle_uss_FOV  = [single(-0.1097),single(-0.9940);single(-0.9940),single(0.1097)];
    %
    Rear_rightRear_uss_FOV  = [single(-0.4602),single(-0.8878);single(-0.8878),single(0.4602)];
    %
    Rear_rightSide_uss_FOV  = [single(-0.9986),single(-0.0523);single(-0.0523),single(0.9986)];
    %
    theta = single(3.141593.*[3/4, 5/8, 1/2, 3/8, 1/4]) ;
    %
    theta_far = single(3.141593.*[5/8, 9/16, 1/2, 7/16, 3/8]);
    %
    theta_side = single(3.141593.*[42/72, 39/72, 36/72, 33/72, 30/72]);
    
    if Sensor_Detection(1) > 0   
        orix = Sensor_Detection(1) * single(cos(theta_side));
        oriy = sqrt(Sensor_Detection(1)^2-orix.^2);
        Longitudial_Dist(:,1) = orix.* Front_leftSide_uss_FOV(1,1) + oriy.*Front_leftSide_uss_FOV(2,1) + Front_leftSide_uss_position_x;
        Lateral_Dist(:,1) = orix.* Front_leftSide_uss_FOV(1,2) + oriy.*Front_leftSide_uss_FOV(2,2) + Front_leftSide_uss_position_y;
    end
    
    if Sensor_Detection(2) > 0  
        if Sensor_Detection(2) <= 600
            orix = Sensor_Detection(2) * cos(theta);
        else
            orix = Sensor_Detection(2) * cos(theta_far);
        end
        oriy = sqrt(Sensor_Detection(2)^2-orix.^2);
        Longitudial_Dist(:,2) = orix.* Front_leftFront_uss_FOV(1,1) + oriy.*Front_leftFront_uss_FOV(2,1) + Front_leftFront_uss_position_x;
        Lateral_Dist(:,2) = orix.* Front_leftFront_uss_FOV(1,2) + oriy.*Front_leftFront_uss_FOV(2,2) + Front_leftFront_uss_position_y;
    end
    
    if Sensor_Detection(3) > 0
        if Sensor_Detection(3) <= 600
            orix = Sensor_Detection(3) * cos(theta);
        else
            orix = Sensor_Detection(3) * cos(theta_far);
        end
        oriy = sqrt(Sensor_Detection(3)^2-orix.^2);
        Longitudial_Dist(:,3) = orix.* Front_leftMiddle_uss_FOV(1,1) + oriy.*Front_leftMiddle_uss_FOV(2,1) + Front_leftMiddle_uss_position_x;
        Lateral_Dist(:,3) = orix.* Front_leftMiddle_uss_FOV(1,2) + oriy.*Front_leftMiddle_uss_FOV(2,2) + Front_leftMiddle_uss_position_y;
    end
    
    if Sensor_Detection(4) > 0
        if Sensor_Detection(4) <= 600
            orix = Sensor_Detection(4) * cos(theta);
        else
            orix = Sensor_Detection(4) * cos(theta_far);
        end
        oriy = sqrt(Sensor_Detection(4)^2-orix.^2);
        Longitudial_Dist(:,4) = orix.* Front_rightMiddle_uss_FOV(1,1) + oriy.*Front_rightMiddle_uss_FOV(2,1) + Front_rightMiddle_uss_position_x;
        Lateral_Dist(:,4) = orix.* Front_rightMiddle_uss_FOV(1,2) + oriy.*Front_rightMiddle_uss_FOV(2,2) + Front_rightMiddle_uss_position_y;
    end
       
    if Sensor_Detection(5) > 0
        if Sensor_Detection(5) <= 600
            orix = Sensor_Detection(5) * cos(theta);
        else
            orix = Sensor_Detection(5) * cos(theta_far);
        end
        oriy = sqrt(Sensor_Detection(5)^2-orix.^2);
        Longitudial_Dist(:,5) = orix.* Front_rightFront_uss_FOV(1,1) + oriy.*Front_rightFront_uss_FOV(2,1) + Front_rightFront_uss_position_x;
        Lateral_Dist(:,5) = orix.* Front_rightFront_uss_FOV(1,2) + oriy.*Front_rightFront_uss_FOV(2,2) + Front_rightFront_uss_position_y;
    end
        
    if Sensor_Detection(6) > 0
        orix = Sensor_Detection(6) * cos(theta_side);
        oriy = sqrt(Sensor_Detection(6)^2-orix.^2);
        Longitudial_Dist(:,6) = orix.* Front_rightSide_uss_FOV(1,1) + oriy.*Front_rightSide_uss_FOV(2,1) + Front_rightSide_uss_position_x;
        Lateral_Dist(:,6) = orix.* Front_rightSide_uss_FOV(1,2) + oriy.*Front_rightSide_uss_FOV(2,2) + Front_rightSide_uss_position_y;
    end
    
    if Sensor_Detection(7) > 0
        orix = Sensor_Detection(7) * cos(theta_side);
        oriy = sqrt(Sensor_Detection(7)^2-orix.^2);
        Longitudial_Dist(:,7) = orix.* Rear_leftSide_uss_FOV(1,1) + oriy.*Rear_leftSide_uss_FOV(2,1) + Rear_leftSide_uss_position_x;
        Lateral_Dist(:,7) = orix.* Rear_leftSide_uss_FOV(1,2) + oriy.*Rear_leftSide_uss_FOV(2,2) + Rear_leftSide_uss_position_y;
    end
    
    if Sensor_Detection(8) > 0
        if Sensor_Detection(8) <= 600
            orix = Sensor_Detection(8) * cos(theta);
        else
            orix = Sensor_Detection(8) * cos(theta_far);
        end
        oriy = sqrt(Sensor_Detection(8)^2-orix.^2);
        Longitudial_Dist(:,8) = orix.* Rear_leftRear_uss_FOV(1,1) + oriy.*Rear_leftRear_uss_FOV(2,1) + Rear_leftRear_uss_position_x;
        Lateral_Dist(:,8) = orix.* Rear_leftRear_uss_FOV(1,2) + oriy.*Rear_leftRear_uss_FOV(2,2) + Rear_leftRear_uss_position_y;
    end
    
    if Sensor_Detection(9) > 0    
        if Sensor_Detection(9) <= 600
            orix = Sensor_Detection(9) * cos(theta);
        else
            orix = Sensor_Detection(9) * cos(theta_far);
        end
        oriy = sqrt(Sensor_Detection(9)^2-orix.^2);
        Longitudial_Dist(:,9) = orix.* Rear_leftMiddle_uss_FOV(1,1) + oriy.*Rear_leftMiddle_uss_FOV(2,1) + Rear_leftMiddle_uss_position_x;
        Lateral_Dist(:,9) = orix.* Rear_leftMiddle_uss_FOV(1,2) + oriy.*Rear_leftMiddle_uss_FOV(2,2) + Rear_leftMiddle_uss_position_y;
    end
        
    if Sensor_Detection(10) > 0
        if Sensor_Detection(10) <= 600
            orix = Sensor_Detection(10) * cos(theta);
        else
            orix = Sensor_Detection(10) * cos(theta_far);
        end
        oriy = sqrt(Sensor_Detection(10)^2-orix.^2);
        Longitudial_Dist(:,10) = orix.* Rear_rightMiddle_uss_FOV(1,1) + oriy.*Rear_rightMiddle_uss_FOV(2,1) + Rear_rightMiddle_uss_position_x;
        Lateral_Dist(:,10) = orix.* Rear_rightMiddle_uss_FOV(1,2) + oriy.*Rear_rightMiddle_uss_FOV(2,2) + Rear_rightMiddle_uss_position_y;
    end
        
    if Sensor_Detection(11) > 0
        if Sensor_Detection(11) <= 600
            orix = Sensor_Detection(11) * cos(theta);
        else
            orix = Sensor_Detection(11) * cos(theta_far);
        end
        oriy = sqrt(Sensor_Detection(11)^2-orix.^2);
        Longitudial_Dist(:,11) = orix.* Rear_rightRear_uss_FOV(1,1) + oriy.*Rear_rightRear_uss_FOV(2,1) + Rear_rightRear_uss_position_x;
        Lateral_Dist(:,11) = orix.* Rear_rightRear_uss_FOV(1,2) + oriy.*Rear_rightRear_uss_FOV(2,2) + Rear_rightRear_uss_position_y;
    end
    
    if Sensor_Detection(12) > 0
        orix = Sensor_Detection(12) * cos(theta_side);
        oriy = sqrt(Sensor_Detection(12)^2-orix.^2);
        Longitudial_Dist(:,12) = orix.* Rear_rightSide_uss_FOV(1,1) + oriy.*Rear_rightSide_uss_FOV(2,1) + Rear_rightSide_uss_position_x;
        Lateral_Dist(:,12) = orix.* Rear_rightSide_uss_FOV(1,2) + oriy.*Rear_rightSide_uss_FOV(2,2) + Rear_rightSide_uss_position_y;
    end
